simulink model "LAB_4"  (R2021a)
settings: Solver=VariableStepAuto  StartTime=0.0  StopTime=10.0  RelTol=1e-3
libraries: simulink x2
settings Model: Creator=MAC  LastModifiedBy=MAC

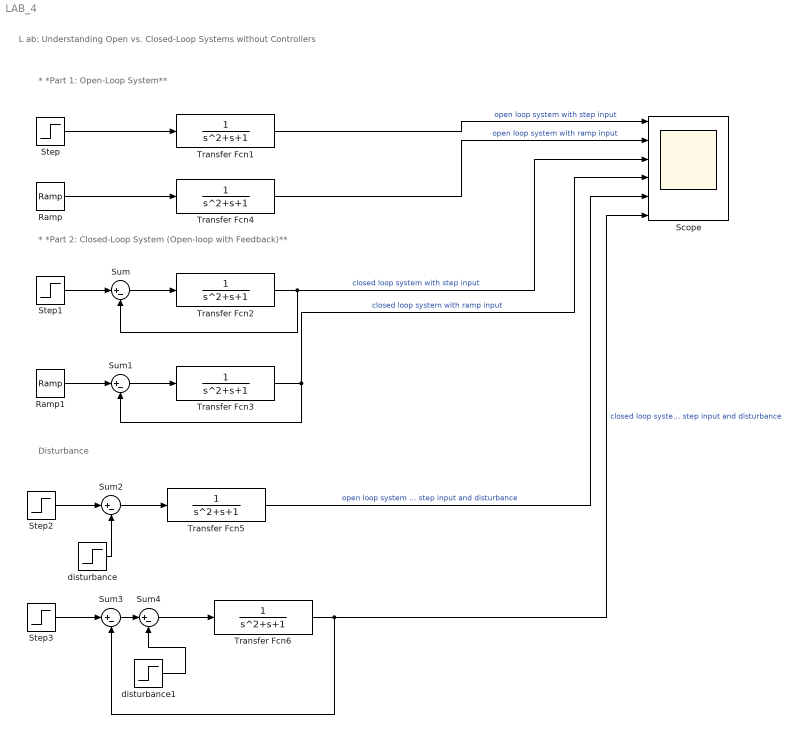
== system LAB_4 ==
  note: Disturbance
  note: * *Part 2: Closed-Loop System (Open-loop with Feedback)**
  note: * *Part 1: Open-Loop System**
  note: L ab: Understanding Open vs. Closed-Loop Systems without Controllers
  Ramp : simulink/Sources/Ramp  slope=1  start=0  InitialOutput=0
  Ramp1 : simulink/Sources/Ramp  slope=1  start=0  InitialOutput=0
  Scope : Scope  NumInputPorts=6
  Step{,1..3} (4 alike) : Step  SampleTime=0
  Sum{,1..4} (5 alike) : Sum  Inputs=|+-
  Transfer Fcn{1..6} (6 alike) : TransferFcn  Denominator=[1 1 1]
  disturbance : Step  Time=5  After=0.2  SampleTime=0
  disturbance1 : Step  Time=5  After=0.2  SampleTime=0
  wires:
  Step/1 -> Transfer Fcn1/1
  Transfer Fcn1/1 -> Scope/1  "open loop system with step input"
  Ramp/1 -> Transfer Fcn4/1
  Transfer Fcn4/1 -> Scope/2  "open loop system with ramp input"
  Transfer Fcn2/1 -> Scope/3, Sum/2  "closed loop system with step input"
  Step1/1 -> Sum/1
  Sum/1 -> Transfer Fcn2/1
  Ramp1/1 -> Sum1/1
  Sum1/1 -> Transfer Fcn3/1
  Transfer Fcn3/1 -> Scope/4, Sum1/2  "closed loop system with ramp input"
  Sum2/1 -> Transfer Fcn5/1
  Step2/1 -> Sum2/1
  disturbance/1 -> Sum2/2
  Transfer Fcn5/1 -> Scope/5  "open loop system with step input and disturbance"
  Step3/1 -> Sum3/1
  Transfer Fcn6/1 -> Scope/6, Sum3/2  "closed loop system with step input and disturbance"
  Sum3/1 -> Sum4/1
  disturbance1/1 -> Sum4/2
  Sum4/1 -> Transfer Fcn6/1
